simulink model "simppend"  (Simulink 7.6)
settings: Solver=ode45  SolverMode=SingleTasking  StartTime=0  StopTime=10000  MaxStep=.1  RelTol=1e-3  AbsTol=1e-6
settings Model: Creator=The MathWorks Inc.  ExtModeAutoUpdateStatusClock=off
settings DataIOCC: ExternalInput=[]  InitialState=[]  LimitDataPoints=off  SaveOutput=off  SaveTime=off
settings OptimizationCC: BlockReduction=off  BooleanDataType=off  InlineInvariantSignals=on  InitFltsAndDblsToZero=on  BufferReusableBoundary=off
settings DebuggingCC: SaveWithParameterizedLinksMsg=none  SignalResolutionControl=TryResolveAllWithWarning  SolverPrmCheckMsg=none  MultiTaskDSMMsg=warning  MultiTaskCondExecSysMsg=none  BusObjectLabelMismatch=none
settings HardwareCC: TargetUnknown=on
settings RTWCC: IncludeERTFirstTime=on
settings GRTTargetCC: TargetFcnLib=ansi_tfl_tmw.mat

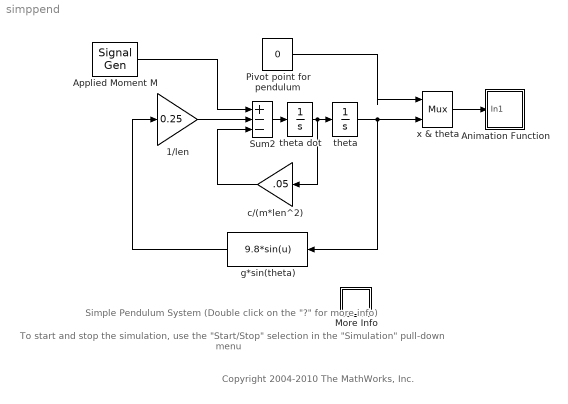
== system simppend ==
  note: Simple Pendulum System
      | (Double click on the "?" for more info)
  note: To start and stop the simulation, use the "Start/Stop"
      | selection in the "Simulation" pull-down menu
  note: Copyright 2004-2010 The MathWorks, Inc.
  1/len : Gain  Gain=0.25  SaturateOnIntegerOverflow=on  OutDataTypeStr=Inherit: Same as input  ParamDataTypeStr=Inherit: Same as input
  Animation Function : Subsystem  mask(Animation Block){ts=0.05}
      mask prompts: ts "Sample time:"
      mask Display: plot([.1,.9],[.9,.9],[.5,.2],[.9,.25],[.475,.475,.525,.525,.475],[.875,.925,.925,.875,.875])
  Applied Moment M : SignalGenerator  WaveForm=square  Frequency=0.100000  Units=rad/sec
  More Info : Subsystem
      mask Display: disp('?')
  Pivot point for pendulum : Constant  Value=0
  Sum2 : Sum  Inputs=+--  SaturateOnIntegerOverflow=on  InputSameDT=on  OutDataTypeStr=Inherit: Same as first input
  c/(m*len^2) : Gain  Gain=.05  SaturateOnIntegerOverflow=on  OutDataTypeStr=Inherit: Same as input  ParamDataTypeStr=Inherit: Same as input
  g*sin(theta) : Fcn  Expr=9.8*sin(u)
  theta : Integrator  InitialCondition=45
  theta dot : Integrator
  x & theta : Mux  Inputs=2
  wires:
  Sum2/1 -> theta dot/1
  c/(m*len^2)/1 -> Sum2/3
  theta dot/1 -> c/(m*len^2)/1, theta/1
  Pivot point for pendulum/1 -> x & theta/1
  theta/1 -> x & theta/2, g*sin(theta)/1
  1/len/1 -> Sum2/2
  g*sin(theta)/1 -> 1/len/1
  Applied Moment M/1 -> Sum2/1
  x & theta/1 -> Animation Function/1(In1)

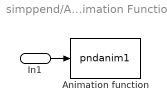
== system simppend/Animation Function ==
  In1 : Inport
  Animation function : S-Function  FunctionName=pndanim1  Parameters=ts  EnableBusSupport=off
      settings: DeleteFcn=shh = get(0,'ShowHiddenHandles');set(0,'ShowHiddenHandles','on');if ~isempty(findobj('type','figure','name','simppend Animation'));close('simppend Animation'); end;set(0,'ShowHiddenHandles',shh);
  wires:
  In1/1 -> Animation function/1

== system simppend/More Info ==
  note: Associated with the demo is an animation function that
      | will automatically open a figure window and display to it.
  note: This system models a simple pendulum system with
      | an applied external moment that varies periodically.
  note: Try experimenting with different initial conditions and
      | different setting for the applied moment M.
